simulink model "SimpleProcess_ExampleIV"  (Simulink 2.20)
settings: Solver=ode4  StartTime=0.0  StopTime=150  FixedStep=0.0025  RelTol=1e-3  AbsTol=1e-6
libraries: DABLib x16
settings Model: ConsistencyChecking=off  RTWPlaceOutputsASAP=off

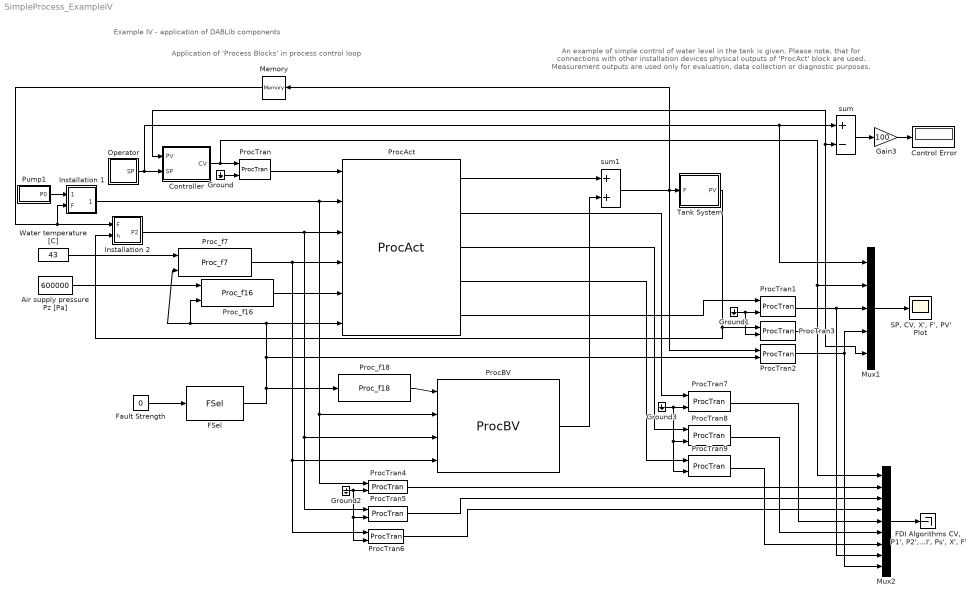
== system SimpleProcess_ExampleIV ==
  note: Application of 'Process Blocks' in process control loop
  note: Example IV - application of DABLib components
  note: An example of simple control of water level in the tank is given.
      | Please note, that for connections with other installation devices physical outputs of 'ProcAct' block are used.
      | Measurement outputs are used only for evaluation, data collection or diagnostic purposes.
  Air supply pressure Pz [Pa] : Constant  Value=600000
  Control Error : Display
      settings: Format=bank  SampleTime=0.1
  Controller : Subsystem  mask(Rozszerzony Regulator PID){P=100, LIMIT=[0 1], ILIMIT=[0 1]}
      mask prompts: P "Proportional:"; LIMIT "Limits:"; ILIMIT "Integration Limits:"
      mask help: CV=min ( LIMIT(2); max( LIMIT(1); (SP-PV)*(1+1/Is+Ds)*P ) )
      mask Display: disp('I')
  "FDI Algorithms CV, P1', P2', T1' Pz', CVI', Ps', X', F'" : Terminator
  FSel : DABLib/FSel  FSel=NO FAULT
  Fault Strength : Constant  Value=0
  Gain3 : Gain  Gain=100
  Ground{,1..3} (4 alike) : Ground
  Installation 1 : Subsystem
  Installation 2 : Subsystem
  Memory : Memory  Orientation=left  X0=0  InheritSampleTime=off
  Mux1 : Mux  Inputs=5
  Mux2 : Mux  Inputs=9
  Operator : Subsystem
  ProcAct : DABLib/ProcessBlk/ProcAct
  ProcBV : DABLib/ProcessBlk/ProcBV
  ProcTran : DABLib/ProcessBlk/ProcTran  ScFact=1  EN=on  Sd=[435435431]  FSel=NO FAULT
  ProcTran1 : DABLib/ProcessBlk/ProcTran  ScFact=1  EN=on  Sd=[43543513]  FSel=NO FAULT
  ProcTran2 : DABLib/ProcessBlk/ProcTran  ScFact=40  EN=on  Sd=[324125]  FSel=f19 - Flow rate sensor fault
  ProcTran3 : DABLib/ProcessBlk/ProcTran  ScFact=2  EN=on  Sd=[568478435]  FSel=NO FAULT
  ProcTran4 : DABLib/ProcessBlk/ProcTran  ScFact=1  EN=on  Sd=[123465]  FSel=NO FAULT
  ProcTran5 : DABLib/ProcessBlk/ProcTran  ScFact=1  EN=on  Sd=[143534565]  FSel=NO FAULT
  ProcTran6 : DABLib/ProcessBlk/ProcTran  ScFact=1  EN=on  Sd=[452543]  FSel=NO FAULT
  ProcTran7 : DABLib/ProcessBlk/ProcTran  ScFact=1  EN=on  Sd=[65487986798]  FSel=NO FAULT
  ProcTran8 : DABLib/ProcessBlk/ProcTran  ScFact=1  EN=on  Sd=[647658748]  FSel=NO FAULT
  ProcTran9 : DABLib/ProcessBlk/ProcTran  ScFact=1  EN=on  Sd=[5465462]  FSel=NO FAULT
  Proc_f16 : DABLib/ProcessBlk/Proc_f16
  Proc_f18 : DABLib/ProcessBlk/Proc_f18
  Proc_f7 : DABLib/ProcessBlk/Proc_f7
  Pump1 : Subsystem
  "SP, CV, X', F', PV' Plot" : Scope
      settings: TickLabels=on  TimeRange=150  YMin=0  YMax=1  SaveToWorkspace=off  SaveName=ScopeData  LimitMaxRows=off
  Tank System : Subsystem
  Water temperature [C] : Constant  Value=43
  sum : Sum  Inputs=+-
  sum1 : Sum  Inputs=2
  wires:
  Fault Strength/1 -> FSel/1
  Pump1/1(P0) -> Installation 1/1(P0)
  Air supply pressure Pz [Pa]/1 -> Proc_f16/1
  Operator/1(SP) -> Controller/2(SP), sum/1, Mux1/1
  Mux1/1 -> "SP, CV, X', F', PV' Plot"/1
  Ground/1 -> ProcTran/2
  Controller/1(CV) -> Mux1/2, Mux2/1, ProcTran/1
  Mux2/1 -> "FDI Algorithms CV, P1', P2', T1' Pz', CVI', Ps', X', F'"/1
  Ground2/1 -> ProcTran4/2, ProcTran5/2, ProcTran6/2
  Ground3/1 -> ProcTran7/2, ProcTran9/2, ProcTran8/2
  Ground1/1 -> ProcTran1/2, ProcTran3/2
  ProcTran7/1 -> Mux2/5
  ProcTran8/1 -> Mux2/6
  ProcTran9/1 -> Mux2/7
  ProcTran1/1 -> Mux1/3, Mux2/8
  sum/1 -> Gain3/1
  Gain3/1 -> Control Error/1
  ProcTran4/1 -> Mux2/2
  ProcTran5/1 -> Mux2/3
  ProcTran6/1 -> Mux2/4
  Installation 1/1(P1) -> ProcAct/2, ProcTran4/1, ProcBV/2
  ProcAct/5 -> ProcTran1/1
  ProcAct/2 -> ProcTran7/1
  ProcAct/3 -> ProcTran8/1
  ProcAct/4 -> ProcTran9/1
  sum1/1 -> Tank System/1(F), ProcTran2/1, Memory/1
  Proc_f18/1 -> ProcBV/1
  ProcTran2/1 -> Mux2/9, Mux1/4
  ProcTran3/1 -> Mux1/5, sum/2, Controller/1(PV)
  ProcAct/1 -> sum1/1
  ProcBV/1 -> sum1/2
  Proc_f16/1 -> ProcAct/5
  Tank System/1(PV) -> ProcTran3/1, Installation 2/2(h)
  Memory/1 -> Installation 2/1(F), Installation 1/2(F)
  ProcTran/1 -> ProcAct/1
  Installation 2/1(P2) -> ProcAct/3, ProcTran5/1, ProcBV/3
  Water temperature [C]/1 -> Proc_f7/1
  Proc_f7/1 -> ProcAct/4, ProcTran6/1, ProcBV/4
  FSel/1 -> Proc_f18/1, ProcAct/6, Proc_f16/2, Proc_f7/2, ProcTran2/2

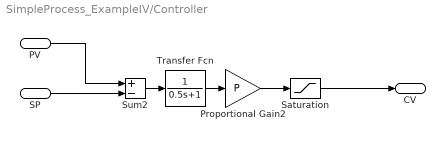
== system SimpleProcess_ExampleIV/Controller ==
  PV : Inport  Port=1  PortWidth=-1  SampleTime=-1
  SP : Inport  Port=2  PortWidth=-1  SampleTime=-1
  Proportional Gain2 : Gain  Gain=P
  Saturation : Saturate  UpperLimit=LIMIT(2)  LowerLimit=LIMIT(1)
  Sum2 : Sum  Inputs=+-
  Transfer Fcn : TransferFcn  Numerator=[1]  Denominator=[0.5 1]
  CV : Outport  Port=1  InitialOutput=0
  wires:
  Saturation/1 -> CV/1
  Proportional Gain2/1 -> Saturation/1
  PV/1 -> Sum2/1
  SP/1 -> Sum2/2
  Sum2/1 -> Transfer Fcn/1
  Transfer Fcn/1 -> Proportional Gain2/1

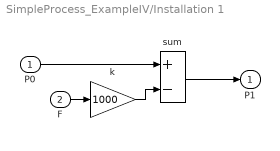
== system SimpleProcess_ExampleIV/Installation 1 ==
  P0 : Inport  Port=1  PortWidth=-1  SampleTime=-1
  F : Inport  Port=2  PortWidth=-1  SampleTime=-1
  k : Gain  Gain=1000
  sum : Sum  Inputs=+-
  P1 : Outport  Port=1  InitialOutput=0
  wires:
  P0/1 -> sum/1
  sum/1 -> P1/1
  F/1 -> k/1
  k/1 -> sum/2

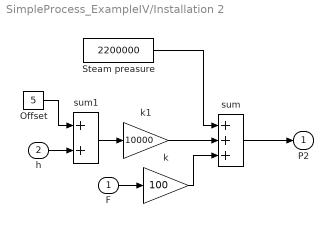
== system SimpleProcess_ExampleIV/Installation 2 ==
  F : Inport  Port=1  PortWidth=-1  SampleTime=-1
  h : Inport  Port=2  PortWidth=-1  SampleTime=-1
  Offset : Constant  Value=5
  Steam preasure : Constant  Value=2200000
  k : Gain  Gain=100
  k1 : Gain  Gain=10000
  sum : Sum  Inputs=3
  sum1 : Sum  Inputs=2
  P2 : Outport  Port=1  InitialOutput=0
  wires:
  sum/1 -> P2/1
  F/1 -> k/1
  h/1 -> sum1/2
  sum1/1 -> k1/1
  Offset/1 -> sum1/1
  Steam preasure/1 -> sum/1
  k1/1 -> sum/2
  k/1 -> sum/3

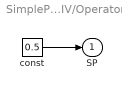
== system SimpleProcess_ExampleIV/Operator ==
  const : Constant  Value=0.5
  SP : Outport  Port=1  InitialOutput=0
  wires:
  const/1 -> SP/1

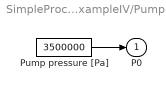
== system SimpleProcess_ExampleIV/Pump1 ==
  "Pump pressure [Pa] " : Constant  Value=3500000
  P0 : Outport  Port=1  InitialOutput=0
  wires:
  "Pump pressure [Pa] "/1 -> P0/1

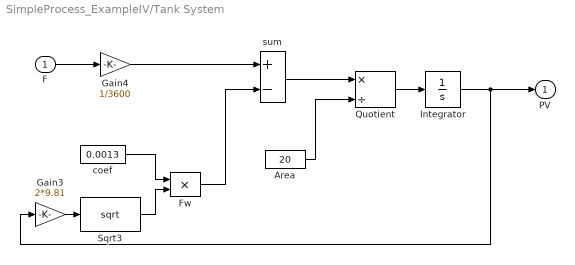
== system SimpleProcess_ExampleIV/Tank System ==
  F : Inport  Port=1  PortWidth=-1  SampleTime=-1
  Area : Constant  Value=20
  Fw : Product  Inputs=2
  Gain3 : Gain  Gain=2*9.81
  Gain4 : Gain  Gain=1/3600
  Integrator : Integrator  ExternalReset=none  InitialConditionSource=internal  InitialCondition=0.9  LimitOutput=on  UpperSaturationLimit=2  LowerSaturationLimit=0  ShowSaturationPort=off  ShowStatePort=off  AbsoluteTolerance=auto
  Quotient : Product  Inputs=*/
  Sqrt3 : MATLABFcn  MATLABFcn=sqrt  OutputWidth=-1
  coef : Constant  Value=0.0013
  sum : Sum  Inputs=+-
  PV : Outport  Port=1  InitialOutput=0
  wires:
  Gain3/1 -> Sqrt3/1
  Sqrt3/1 -> Fw/2
  coef/1 -> Fw/1
  Quotient/1 -> Integrator/1
  sum/1 -> Quotient/1
  Area/1 -> Quotient/2
  Integrator/1 -> PV/1, Gain3/1
  F/1 -> Gain4/1
  Gain4/1 -> sum/1
  Fw/1 -> sum/2
